simulink model "tank-model-lookup"  (R2018a)
settings: Solver=FixedStepAuto  StartTime=0.0  StopTime=10  FixedStep=.1  RelTol=1e-3  EnableMultiTasking=on
settings Model: Creator=gwilfong  LastModifiedBy=gwilfong
settings DataIOCC: LimitDataPoints=on  SaveFormat=Array
settings OptimizationCC: LifeSpan=inf
settings DebuggingCC: SFUnexpectedBacktrackingDiag=warning  SFNoUnconditionalDefaultTransitionDiag=warning  SFExecutionAtInitializationDiag=none
settings HardwareCC: ProdBitPerPointer=32  ProdBitPerSizeT=32  ProdBitPerPtrDiffT=32  ProdLargestAtomicFloat=None  ProdIntDivRoundTo=Undefined  ProdEndianess=Unspecified  ProdWordSize=32  ProdHWDeviceType=32-bit Generic
settings ModelReferenceCC: PropagateSignalLabelsOutOfModel=off
settings CodeAppCC: StateflowObjectComments=on
settings GRTTargetCC: TargetLangStandard=C89/C90 (ANSI)  GeneratePreprocessorConditionals=Disable all
settings ConfigComp: CovMetricSettings=dw  CovHtmlReporting=on  CovSaveCumulativeToWorkspaceVar=on  CovSaveSingleToWorkspaceVar=on  CovExternalEMLEnable=off

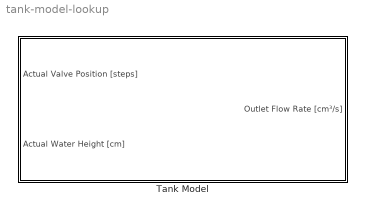
== system tank-model-lookup ==
  Tank Model : Subsystem

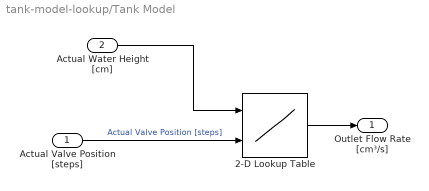
== system tank-model-lookup/Tank Model ==
  Actual Valve Position [steps] : Inport
  Actual Water Height [cm] : Inport  Port=2
  2-D Lookup Table : Lookup_n-D  BreakpointsForDimension1=[7 8 9 10 11 12 13 14 15 16 17 18 19 20 21 22 23 24 25 26 27 28 29 30 31]  BreakpointsForDimension2=[0 100 200 300 400 600 800 1020]  Table=[0 -16.41851658 -80.88721297 -157.949763 -307.0263376 -480.4515967 -628.0110768 -741.5526829;0 -16.61601261 -81.8602152 -159.8503252 -310.7215641 -486.2346651 -635.5697772 -750.4747526; 0 -16.81456354 -82.83840749 -161.7609182 -314.4361873 -492.0480213 -643.1680547 -759.444035; 0 -17.01416938 -83.82178983 -163.6815421 -318.170207 -497.8916652 -650.8059094 -768.4605302; 0 -17.21483012 -84.81036222 -165.6121969 -321.9236234 -503.7655969 -658.4833411 -777.5242381; 0 -17.41654577 -85.80412465 -167.5528826 -325.6964365 -509.6698163 -666.20035 -786.6351588; 0 -17.61931632 -86.80307714 -169.5035992 -329.4886461 -515.6043234 -673.956936 -795.7932923; 0 -17.82314178 -87.80721968 -171.4643466 -333.3002524 -521.5691183 -681.7530992 -804.9986385; 0 -18.02802214 -88.81655227 -173.4351249 -337.1312554 -527.564201 -689.5888394 -814.2511974; 0 -18.2339574 -89.83107492 -175.4159341 -340.9816549 -533.5895713 -697.4641568 -823.5509692; 0 -18.44094757 -90.85078761 -177.4067742 -344.8514511 -539.6452295 -705.3790513 -832.8979536; 0 -18.64899265 -91.87569035 -179.4076451 -348.7406439 -545.7311753 -713.333523 -842.2921509; 0 -18.85809263 -92.90578314 -181.4185469 -352.6492334 -551.8474089 -721.3275718 -851.7335608; 0 -19.06824751 -93.94106599 -183.4394796 -356.5772195 -557.9939303 -729.3611976 -861.2221836; 0 -19.2794573 -94.98153888 -185.4704432 -360.5246022 -564.1707394 -737.4344007 -870.7580191; 0 -19.49172199 -96.02720183 -187.5114376 -364.4913816 -570.3778362 -745.5471808 -880.3410673; 0 -19.70504159 -97.07805482 -189.562463 -368.4775576 -576.6152208 -753.6995381 -889.9713283; 0 -19.91941609 -98.13409787 -191.6235192 -372.4831302 -582.8828931 -761.8914725 -899.6488021; 0 -20.1348455 -99.19533097 -193.6946062 -376.5080994 -589.1808532 -770.122984 -909.3734886; 0 -20.35132981 -100.2617541 -195.7757242 -380.5524653 -595.509101 -778.3940726 -919.1453879; 0 -20.56886902 -101.3333673 -197.866873 -384.6162279 -601.8676365 -786.7047384 -928.9644999; 0 -20.78746314 -102.4101706 -199.9680528 -388.699387 -608.2564598 -795.0549813 -938.8308247; 0 -21.00711217 -103.4921639 -202.0792633 -392.8019428 -614.6755708 -803.4448013 -948.7443622; 0 -21.2278161 -104.5793472 -204.2005048 -396.9238952 -621.1249696 -811.8741984 -958.7051125; 0 -21.44957493 -105.6717206 -206.3317772 -401.0652443 -627.6046561 -820.3431727 -968.7130756]  InternalRulePriority=Speed  RndMeth=Simplest  InputSameDT=on
  Outlet Flow Rate [cm³/s] : Outport
  wires:
  Actual Valve Position [steps]/1 -> 2-D Lookup Table/2  "Actual Valve Position [steps]"
  2-D Lookup Table/1 -> Outlet Flow Rate [cm³/s]/1
  Actual Water Height [cm]/1 -> 2-D Lookup Table/1
